simulink subsystem "station2a"  (R2024b)
settings: Solver=VariableStepAuto  StartTime=0.0  StopTime=10.0  RelTol=1e-3
undefined symbols (not defined in the file): DiscIntNeverNeededParam, h, R3, ResistanceM, Rt4, Ts, Zm
libraries: fl_lib x239, ee_lib x102, nesl_utility x83, simulink x6, simetran x1, powerlib_extras x1
(part 5 of 5)

== system station2a/Filters 60Hz5/tuned filter 13th ==
  Electrical Reference : fl_lib/Electrical/Electrical Elements/Electrical Reference
  Electrical Reference1 : fl_lib/Electrical/Electrical Elements/Electrical Reference
  Electrical Reference2 : fl_lib/Electrical/Electrical Elements/Electrical Reference
  Inductor : fl_lib/Electrical/Electrical Elements/Inductor  l=L1 H  r=R2 Ohm  g=1e-9 1/Ohm  i_specify=off  i_priority=None  i=0 A  i_nominal_specify=off  i_nominal_value=1  i_nominal_unit=A  v_specify=off  v_priority=None  v=0 V  v_nominal_specify=off  v_nominal_value=1  v_nominal_unit=V  i_L_specify=off  i_L_priority=High  i_L=0 A  i_L_nominal_specify=off  i_L_nominal_value=1  i_L_nominal_unit=A
  Inductor1 : fl_lib/Electrical/Electrical Elements/Inductor  l=L1 H  r=R2 Ohm  g=1e-9 1/Ohm  i_specify=off  i_priority=None  i=0 A  i_nominal_specify=off  i_nominal_value=1  i_nominal_unit=A  v_specify=off  v_priority=None  v=0 V  v_nominal_specify=off  v_nominal_value=1  v_nominal_unit=V  i_L_specify=off  i_L_priority=High  i_L=0 A  i_L_nominal_specify=off  i_L_nominal_value=1  i_L_nominal_unit=A
  Inductor2 : fl_lib/Electrical/Electrical Elements/Inductor  l=L1 H  r=R2 Ohm  g=1e-9 1/Ohm  i_specify=off  i_priority=None  i=0 A  i_nominal_specify=off  i_nominal_value=1  i_nominal_unit=A  v_specify=off  v_priority=None  v=0 V  v_nominal_specify=off  v_nominal_value=1  v_nominal_unit=V  i_L_specify=off  i_L_priority=High  i_L=0 A  i_L_nominal_specify=off  i_L_nominal_value=1  i_L_nominal_unit=A
  Phase Splitter : ee_lib/Connectors & References/Phase Splitter
  RC : fl_lib/Electrical/Electrical Elements/Capacitor  c=C1 F  r=0 Ohm  g=0 1/Ohm  i_specify=off  i_priority=None  i=0 A  i_nominal_specify=off  i_nominal_value=1  i_nominal_unit=A  v_specify=off  v_priority=None  v=0 V  v_nominal_specify=off  v_nominal_value=1  v_nominal_unit=V  vc_specify=off  vc_priority=High  vc=0 V  vc_nominal_specify=off  vc_nominal_value=1  vc_nominal_unit=V
  RC1 : fl_lib/Electrical/Electrical Elements/Capacitor  c=C1 F  r=0 Ohm  g=0 1/Ohm  i_specify=off  i_priority=None  i=0 A  i_nominal_specify=off  i_nominal_value=1  i_nominal_unit=A  v_specify=off  v_priority=None  v=0 V  v_nominal_specify=off  v_nominal_value=1  v_nominal_unit=V  vc_specify=off  vc_priority=High  vc=0 V  vc_nominal_specify=off  vc_nominal_value=1  vc_nominal_unit=V
  RC2 : fl_lib/Electrical/Electrical Elements/Capacitor  c=C1 F  r=0 Ohm  g=0 1/Ohm  i_specify=off  i_priority=None  i=0 A  i_nominal_specify=off  i_nominal_value=1  i_nominal_unit=A  v_specify=off  v_priority=None  v=0 V  v_nominal_specify=off  v_nominal_value=1  v_nominal_unit=V  vc_specify=off  vc_priority=High  vc=0 V  vc_nominal_specify=off  vc_nominal_value=1  vc_nominal_unit=V
  abc : PMIOPort  Side=Right
  connections:
  Inductor/LConn1 -- RC/RConn1
  Inductor/RConn1 -- Electrical Reference/LConn1
  RC1/RConn1 -- Inductor1/LConn1
  Inductor1/RConn1 -- Electrical Reference1/LConn1
  Inductor2/RConn1 -- Electrical Reference2/LConn1
  RC2/RConn1 -- Inductor2/LConn1
  Phase Splitter/RConn2 -- RC1/LConn1
  RC/LConn1 -- Phase Splitter/RConn1
  RC2/LConn1 -- Phase Splitter/RConn3
  Phase Splitter/LConn1 -- abc/RConn1

== system station2a/Filters 60Hz6/High-pass filter ==
  CC : fl_lib/Electrical/Electrical Elements/Capacitor  c=C1 F  r=0 Ohm  g=0 1/Ohm  i_specify=off  i_priority=None  i=0 A  i_nominal_specify=off  i_nominal_value=1  i_nominal_unit=A  v_specify=off  v_priority=None  v=0 V  v_nominal_specify=off  v_nominal_value=1  v_nominal_unit=V  vc_specify=off  vc_priority=High  vc=0 V  vc_nominal_specify=off  vc_nominal_value=1  vc_nominal_unit=V
  CC1 : fl_lib/Electrical/Electrical Elements/Capacitor  c=C1 F  r=0 Ohm  g=0 1/Ohm  i_specify=off  i_priority=None  i=0 A  i_nominal_specify=off  i_nominal_value=1  i_nominal_unit=A  v_specify=off  v_priority=None  v=0 V  v_nominal_specify=off  v_nominal_value=1  v_nominal_unit=V  vc_specify=off  vc_priority=High  vc=0 V  vc_nominal_specify=off  vc_nominal_value=1  vc_nominal_unit=V
  CC2 : fl_lib/Electrical/Electrical Elements/Capacitor  c=C1 F  r=0 Ohm  g=0 1/Ohm  i_specify=off  i_priority=None  i=0 A  i_nominal_specify=off  i_nominal_value=1  i_nominal_unit=A  v_specify=off  v_priority=None  v=0 V  v_nominal_specify=off  v_nominal_value=1  v_nominal_unit=V  vc_specify=off  vc_priority=High  vc=0 V  vc_nominal_specify=off  vc_nominal_value=1  vc_nominal_unit=V
  Electrical Reference : fl_lib/Electrical/Electrical Elements/Electrical Reference
  Electrical Reference1 : fl_lib/Electrical/Electrical Elements/Electrical Reference
  Electrical Reference2 : fl_lib/Electrical/Electrical Elements/Electrical Reference
  Phase Splitter : ee_lib/Connectors & References/Phase Splitter
  RL parallel : fl_lib/Electrical/Electrical Elements/Inductor  l=L2 H  r=0 Ohm  g=1/R3 1/Ohm  i_specify=off  i_priority=None  i=0 A  i_nominal_specify=off  i_nominal_value=1  i_nominal_unit=A  v_specify=off  v_priority=None  v=0 V  v_nominal_specify=off  v_nominal_value=1  v_nominal_unit=V  i_L_specify=off  i_L_priority=High  i_L=0 A  i_L_nominal_specify=off  i_L_nominal_value=1  i_L_nominal_unit=A
  RL parallel1 : fl_lib/Electrical/Electrical Elements/Inductor  l=L2 H  r=0 Ohm  g=1/R3 1/Ohm  i_specify=off  i_priority=None  i=0 A  i_nominal_specify=off  i_nominal_value=1  i_nominal_unit=A  v_specify=off  v_priority=None  v=0 V  v_nominal_specify=off  v_nominal_value=1  v_nominal_unit=V  i_L_specify=off  i_L_priority=High  i_L=0 A  i_L_nominal_specify=off  i_L_nominal_value=1  i_L_nominal_unit=A
  RL parallel2 : fl_lib/Electrical/Electrical Elements/Inductor  l=L2 H  r=0 Ohm  g=1/R3 1/Ohm  i_specify=off  i_priority=None  i=0 A  i_nominal_specify=off  i_nominal_value=1  i_nominal_unit=A  v_specify=off  v_priority=None  v=0 V  v_nominal_specify=off  v_nominal_value=1  v_nominal_unit=V  i_L_specify=off  i_L_priority=High  i_L=0 A  i_L_nominal_specify=off  i_L_nominal_value=1  i_L_nominal_unit=A
  abc : PMIOPort  Side=Right
  connections:
  CC2/RConn1 -- RL parallel2/LConn1
  RL parallel2/RConn1 -- Electrical Reference2/LConn1
  RL parallel1/RConn1 -- Electrical Reference1/LConn1
  CC1/RConn1 -- RL parallel1/LConn1
  RL parallel/RConn1 -- Electrical Reference/LConn1
  RL parallel/LConn1 -- CC/RConn1
  Phase Splitter/LConn1 -- abc/RConn1
  Phase Splitter/RConn2 -- CC1/LConn1
  CC/LConn1 -- Phase Splitter/RConn1
  CC2/LConn1 -- Phase Splitter/RConn3

== system station2a/Filters 60Hz6/tuned filter 11th ==
  Electrical Reference : fl_lib/Electrical/Electrical Elements/Electrical Reference
  Electrical Reference1 : fl_lib/Electrical/Electrical Elements/Electrical Reference
  Electrical Reference2 : fl_lib/Electrical/Electrical Elements/Electrical Reference
  Inductor : fl_lib/Electrical/Electrical Elements/Inductor  l=L1 H  r=R2 Ohm  g=1e-9 1/Ohm  i_specify=off  i_priority=None  i=0 A  i_nominal_specify=off  i_nominal_value=1  i_nominal_unit=A  v_specify=off  v_priority=None  v=0 V  v_nominal_specify=off  v_nominal_value=1  v_nominal_unit=V  i_L_specify=off  i_L_priority=High  i_L=0 A  i_L_nominal_specify=off  i_L_nominal_value=1  i_L_nominal_unit=A
  Inductor1 : fl_lib/Electrical/Electrical Elements/Inductor  l=L1 H  r=R2 Ohm  g=1e-9 1/Ohm  i_specify=off  i_priority=None  i=0 A  i_nominal_specify=off  i_nominal_value=1  i_nominal_unit=A  v_specify=off  v_priority=None  v=0 V  v_nominal_specify=off  v_nominal_value=1  v_nominal_unit=V  i_L_specify=off  i_L_priority=High  i_L=0 A  i_L_nominal_specify=off  i_L_nominal_value=1  i_L_nominal_unit=A
  Inductor2 : fl_lib/Electrical/Electrical Elements/Inductor  l=L1 H  r=R2 Ohm  g=1e-9 1/Ohm  i_specify=off  i_priority=None  i=0 A  i_nominal_specify=off  i_nominal_value=1  i_nominal_unit=A  v_specify=off  v_priority=None  v=0 V  v_nominal_specify=off  v_nominal_value=1  v_nominal_unit=V  i_L_specify=off  i_L_priority=High  i_L=0 A  i_L_nominal_specify=off  i_L_nominal_value=1  i_L_nominal_unit=A
  Phase Splitter : ee_lib/Connectors & References/Phase Splitter
  RC : fl_lib/Electrical/Electrical Elements/Capacitor  c=C1 F  r=0 Ohm  g=0 1/Ohm  i_specify=off  i_priority=None  i=0 A  i_nominal_specify=off  i_nominal_value=1  i_nominal_unit=A  v_specify=off  v_priority=None  v=0 V  v_nominal_specify=off  v_nominal_value=1  v_nominal_unit=V  vc_specify=off  vc_priority=High  vc=0 V  vc_nominal_specify=off  vc_nominal_value=1  vc_nominal_unit=V
  RC1 : fl_lib/Electrical/Electrical Elements/Capacitor  c=C1 F  r=0 Ohm  g=0 1/Ohm  i_specify=off  i_priority=None  i=0 A  i_nominal_specify=off  i_nominal_value=1  i_nominal_unit=A  v_specify=off  v_priority=None  v=0 V  v_nominal_specify=off  v_nominal_value=1  v_nominal_unit=V  vc_specify=off  vc_priority=High  vc=0 V  vc_nominal_specify=off  vc_nominal_value=1  vc_nominal_unit=V
  RC2 : fl_lib/Electrical/Electrical Elements/Capacitor  c=C1 F  r=0 Ohm  g=0 1/Ohm  i_specify=off  i_priority=None  i=0 A  i_nominal_specify=off  i_nominal_value=1  i_nominal_unit=A  v_specify=off  v_priority=None  v=0 V  v_nominal_specify=off  v_nominal_value=1  v_nominal_unit=V  vc_specify=off  vc_priority=High  vc=0 V  vc_nominal_specify=off  vc_nominal_value=1  vc_nominal_unit=V
  abc : PMIOPort  Side=Right
  connections:
  Inductor/LConn1 -- RC/RConn1
  Inductor/RConn1 -- Electrical Reference/LConn1
  RC1/RConn1 -- Inductor1/LConn1
  Inductor1/RConn1 -- Electrical Reference1/LConn1
  Inductor2/RConn1 -- Electrical Reference2/LConn1
  RC2/RConn1 -- Inductor2/LConn1
  Phase Splitter/RConn2 -- RC1/LConn1
  RC/LConn1 -- Phase Splitter/RConn1
  RC2/LConn1 -- Phase Splitter/RConn3
  Phase Splitter/LConn1 -- abc/RConn1

== system station2a/Filters 60Hz6/tuned filter 13th ==
  Electrical Reference : fl_lib/Electrical/Electrical Elements/Electrical Reference
  Electrical Reference1 : fl_lib/Electrical/Electrical Elements/Electrical Reference
  Electrical Reference2 : fl_lib/Electrical/Electrical Elements/Electrical Reference
  Inductor : fl_lib/Electrical/Electrical Elements/Inductor  l=L1 H  r=R2 Ohm  g=1e-9 1/Ohm  i_specify=off  i_priority=None  i=0 A  i_nominal_specify=off  i_nominal_value=1  i_nominal_unit=A  v_specify=off  v_priority=None  v=0 V  v_nominal_specify=off  v_nominal_value=1  v_nominal_unit=V  i_L_specify=off  i_L_priority=High  i_L=0 A  i_L_nominal_specify=off  i_L_nominal_value=1  i_L_nominal_unit=A
  Inductor1 : fl_lib/Electrical/Electrical Elements/Inductor  l=L1 H  r=R2 Ohm  g=1e-9 1/Ohm  i_specify=off  i_priority=None  i=0 A  i_nominal_specify=off  i_nominal_value=1  i_nominal_unit=A  v_specify=off  v_priority=None  v=0 V  v_nominal_specify=off  v_nominal_value=1  v_nominal_unit=V  i_L_specify=off  i_L_priority=High  i_L=0 A  i_L_nominal_specify=off  i_L_nominal_value=1  i_L_nominal_unit=A
  Inductor2 : fl_lib/Electrical/Electrical Elements/Inductor  l=L1 H  r=R2 Ohm  g=1e-9 1/Ohm  i_specify=off  i_priority=None  i=0 A  i_nominal_specify=off  i_nominal_value=1  i_nominal_unit=A  v_specify=off  v_priority=None  v=0 V  v_nominal_specify=off  v_nominal_value=1  v_nominal_unit=V  i_L_specify=off  i_L_priority=High  i_L=0 A  i_L_nominal_specify=off  i_L_nominal_value=1  i_L_nominal_unit=A
  Phase Splitter : ee_lib/Connectors & References/Phase Splitter
  RC : fl_lib/Electrical/Electrical Elements/Capacitor  c=C1 F  r=0 Ohm  g=0 1/Ohm  i_specify=off  i_priority=None  i=0 A  i_nominal_specify=off  i_nominal_value=1  i_nominal_unit=A  v_specify=off  v_priority=None  v=0 V  v_nominal_specify=off  v_nominal_value=1  v_nominal_unit=V  vc_specify=off  vc_priority=High  vc=0 V  vc_nominal_specify=off  vc_nominal_value=1  vc_nominal_unit=V
  RC1 : fl_lib/Electrical/Electrical Elements/Capacitor  c=C1 F  r=0 Ohm  g=0 1/Ohm  i_specify=off  i_priority=None  i=0 A  i_nominal_specify=off  i_nominal_value=1  i_nominal_unit=A  v_specify=off  v_priority=None  v=0 V  v_nominal_specify=off  v_nominal_value=1  v_nominal_unit=V  vc_specify=off  vc_priority=High  vc=0 V  vc_nominal_specify=off  vc_nominal_value=1  vc_nominal_unit=V
  RC2 : fl_lib/Electrical/Electrical Elements/Capacitor  c=C1 F  r=0 Ohm  g=0 1/Ohm  i_specify=off  i_priority=None  i=0 A  i_nominal_specify=off  i_nominal_value=1  i_nominal_unit=A  v_specify=off  v_priority=None  v=0 V  v_nominal_specify=off  v_nominal_value=1  v_nominal_unit=V  vc_specify=off  vc_priority=High  vc=0 V  vc_nominal_specify=off  vc_nominal_value=1  vc_nominal_unit=V
  abc : PMIOPort  Side=Right
  connections:
  Phase Splitter/LConn1 -- abc/RConn1
  RC2/LConn1 -- Phase Splitter/RConn3
  RC/LConn1 -- Phase Splitter/RConn1
  Phase Splitter/RConn2 -- RC1/LConn1
  RC2/RConn1 -- Inductor2/LConn1
  Inductor2/RConn1 -- Electrical Reference2/LConn1
  Inductor1/RConn1 -- Electrical Reference1/LConn1
  RC1/RConn1 -- Inductor1/LConn1
  Inductor/RConn1 -- Electrical Reference/LConn1
  Inductor/LConn1 -- RC/RConn1

== system station2a/Filters 60Hz7/High-pass filter ==
  CC : fl_lib/Electrical/Electrical Elements/Capacitor  c=C1 F  r=0 Ohm  g=0 1/Ohm  i_specify=off  i_priority=None  i=0 A  i_nominal_specify=off  i_nominal_value=1  i_nominal_unit=A  v_specify=off  v_priority=None  v=0 V  v_nominal_specify=off  v_nominal_value=1  v_nominal_unit=V  vc_specify=off  vc_priority=High  vc=0 V  vc_nominal_specify=off  vc_nominal_value=1  vc_nominal_unit=V
  CC1 : fl_lib/Electrical/Electrical Elements/Capacitor  c=C1 F  r=0 Ohm  g=0 1/Ohm  i_specify=off  i_priority=None  i=0 A  i_nominal_specify=off  i_nominal_value=1  i_nominal_unit=A  v_specify=off  v_priority=None  v=0 V  v_nominal_specify=off  v_nominal_value=1  v_nominal_unit=V  vc_specify=off  vc_priority=High  vc=0 V  vc_nominal_specify=off  vc_nominal_value=1  vc_nominal_unit=V
  CC2 : fl_lib/Electrical/Electrical Elements/Capacitor  c=C1 F  r=0 Ohm  g=0 1/Ohm  i_specify=off  i_priority=None  i=0 A  i_nominal_specify=off  i_nominal_value=1  i_nominal_unit=A  v_specify=off  v_priority=None  v=0 V  v_nominal_specify=off  v_nominal_value=1  v_nominal_unit=V  vc_specify=off  vc_priority=High  vc=0 V  vc_nominal_specify=off  vc_nominal_value=1  vc_nominal_unit=V
  Electrical Reference : fl_lib/Electrical/Electrical Elements/Electrical Reference
  Electrical Reference1 : fl_lib/Electrical/Electrical Elements/Electrical Reference
  Electrical Reference2 : fl_lib/Electrical/Electrical Elements/Electrical Reference
  Phase Splitter : ee_lib/Connectors & References/Phase Splitter
  RL parallel : fl_lib/Electrical/Electrical Elements/Inductor  l=L2 H  r=0 Ohm  g=1/R3 1/Ohm  i_specify=off  i_priority=None  i=0 A  i_nominal_specify=off  i_nominal_value=1  i_nominal_unit=A  v_specify=off  v_priority=None  v=0 V  v_nominal_specify=off  v_nominal_value=1  v_nominal_unit=V  i_L_specify=off  i_L_priority=High  i_L=0 A  i_L_nominal_specify=off  i_L_nominal_value=1  i_L_nominal_unit=A
  RL parallel1 : fl_lib/Electrical/Electrical Elements/Inductor  l=L2 H  r=0 Ohm  g=1/R3 1/Ohm  i_specify=off  i_priority=None  i=0 A  i_nominal_specify=off  i_nominal_value=1  i_nominal_unit=A  v_specify=off  v_priority=None  v=0 V  v_nominal_specify=off  v_nominal_value=1  v_nominal_unit=V  i_L_specify=off  i_L_priority=High  i_L=0 A  i_L_nominal_specify=off  i_L_nominal_value=1  i_L_nominal_unit=A
  RL parallel2 : fl_lib/Electrical/Electrical Elements/Inductor  l=L2 H  r=0 Ohm  g=1/R3 1/Ohm  i_specify=off  i_priority=None  i=0 A  i_nominal_specify=off  i_nominal_value=1  i_nominal_unit=A  v_specify=off  v_priority=None  v=0 V  v_nominal_specify=off  v_nominal_value=1  v_nominal_unit=V  i_L_specify=off  i_L_priority=High  i_L=0 A  i_L_nominal_specify=off  i_L_nominal_value=1  i_L_nominal_unit=A
  abc : PMIOPort  Side=Right
  connections:
  CC2/LConn1 -- Phase Splitter/RConn3
  CC/LConn1 -- Phase Splitter/RConn1
  Phase Splitter/RConn2 -- CC1/LConn1
  Phase Splitter/LConn1 -- abc/RConn1
  RL parallel/LConn1 -- CC/RConn1
  RL parallel/RConn1 -- Electrical Reference/LConn1
  CC1/RConn1 -- RL parallel1/LConn1
  RL parallel1/RConn1 -- Electrical Reference1/LConn1
  RL parallel2/RConn1 -- Electrical Reference2/LConn1
  CC2/RConn1 -- RL parallel2/LConn1

== system station2a/Filters 60Hz7/tuned filter 11th ==
  Electrical Reference : fl_lib/Electrical/Electrical Elements/Electrical Reference
  Electrical Reference1 : fl_lib/Electrical/Electrical Elements/Electrical Reference
  Electrical Reference2 : fl_lib/Electrical/Electrical Elements/Electrical Reference
  Inductor : fl_lib/Electrical/Electrical Elements/Inductor  l=L1 H  r=R2 Ohm  g=1e-9 1/Ohm  i_specify=off  i_priority=None  i=0 A  i_nominal_specify=off  i_nominal_value=1  i_nominal_unit=A  v_specify=off  v_priority=None  v=0 V  v_nominal_specify=off  v_nominal_value=1  v_nominal_unit=V  i_L_specify=off  i_L_priority=High  i_L=0 A  i_L_nominal_specify=off  i_L_nominal_value=1  i_L_nominal_unit=A
  Inductor1 : fl_lib/Electrical/Electrical Elements/Inductor  l=L1 H  r=R2 Ohm  g=1e-9 1/Ohm  i_specify=off  i_priority=None  i=0 A  i_nominal_specify=off  i_nominal_value=1  i_nominal_unit=A  v_specify=off  v_priority=None  v=0 V  v_nominal_specify=off  v_nominal_value=1  v_nominal_unit=V  i_L_specify=off  i_L_priority=High  i_L=0 A  i_L_nominal_specify=off  i_L_nominal_value=1  i_L_nominal_unit=A
  Inductor2 : fl_lib/Electrical/Electrical Elements/Inductor  l=L1 H  r=R2 Ohm  g=1e-9 1/Ohm  i_specify=off  i_priority=None  i=0 A  i_nominal_specify=off  i_nominal_value=1  i_nominal_unit=A  v_specify=off  v_priority=None  v=0 V  v_nominal_specify=off  v_nominal_value=1  v_nominal_unit=V  i_L_specify=off  i_L_priority=High  i_L=0 A  i_L_nominal_specify=off  i_L_nominal_value=1  i_L_nominal_unit=A
  Phase Splitter : ee_lib/Connectors & References/Phase Splitter
  RC : fl_lib/Electrical/Electrical Elements/Capacitor  c=C1 F  r=0 Ohm  g=0 1/Ohm  i_specify=off  i_priority=None  i=0 A  i_nominal_specify=off  i_nominal_value=1  i_nominal_unit=A  v_specify=off  v_priority=None  v=0 V  v_nominal_specify=off  v_nominal_value=1  v_nominal_unit=V  vc_specify=off  vc_priority=High  vc=0 V  vc_nominal_specify=off  vc_nominal_value=1  vc_nominal_unit=V
  RC1 : fl_lib/Electrical/Electrical Elements/Capacitor  c=C1 F  r=0 Ohm  g=0 1/Ohm  i_specify=off  i_priority=None  i=0 A  i_nominal_specify=off  i_nominal_value=1  i_nominal_unit=A  v_specify=off  v_priority=None  v=0 V  v_nominal_specify=off  v_nominal_value=1  v_nominal_unit=V  vc_specify=off  vc_priority=High  vc=0 V  vc_nominal_specify=off  vc_nominal_value=1  vc_nominal_unit=V
  RC2 : fl_lib/Electrical/Electrical Elements/Capacitor  c=C1 F  r=0 Ohm  g=0 1/Ohm  i_specify=off  i_priority=None  i=0 A  i_nominal_specify=off  i_nominal_value=1  i_nominal_unit=A  v_specify=off  v_priority=None  v=0 V  v_nominal_specify=off  v_nominal_value=1  v_nominal_unit=V  vc_specify=off  vc_priority=High  vc=0 V  vc_nominal_specify=off  vc_nominal_value=1  vc_nominal_unit=V
  abc : PMIOPort  Side=Right
  connections:
  Phase Splitter/LConn1 -- abc/RConn1
  RC2/LConn1 -- Phase Splitter/RConn3
  RC/LConn1 -- Phase Splitter/RConn1
  Phase Splitter/RConn2 -- RC1/LConn1
  RC2/RConn1 -- Inductor2/LConn1
  Inductor2/RConn1 -- Electrical Reference2/LConn1
  Inductor1/RConn1 -- Electrical Reference1/LConn1
  RC1/RConn1 -- Inductor1/LConn1
  Inductor/RConn1 -- Electrical Reference/LConn1
  Inductor/LConn1 -- RC/RConn1

== system station2a/Filters 60Hz7/tuned filter 13th ==
  Electrical Reference : fl_lib/Electrical/Electrical Elements/Electrical Reference
  Electrical Reference1 : fl_lib/Electrical/Electrical Elements/Electrical Reference
  Electrical Reference2 : fl_lib/Electrical/Electrical Elements/Electrical Reference
  Inductor : fl_lib/Electrical/Electrical Elements/Inductor  l=L1 H  r=R2 Ohm  g=1e-9 1/Ohm  i_specify=off  i_priority=None  i=0 A  i_nominal_specify=off  i_nominal_value=1  i_nominal_unit=A  v_specify=off  v_priority=None  v=0 V  v_nominal_specify=off  v_nominal_value=1  v_nominal_unit=V  i_L_specify=off  i_L_priority=High  i_L=0 A  i_L_nominal_specify=off  i_L_nominal_value=1  i_L_nominal_unit=A
  Inductor1 : fl_lib/Electrical/Electrical Elements/Inductor  l=L1 H  r=R2 Ohm  g=1e-9 1/Ohm  i_specify=off  i_priority=None  i=0 A  i_nominal_specify=off  i_nominal_value=1  i_nominal_unit=A  v_specify=off  v_priority=None  v=0 V  v_nominal_specify=off  v_nominal_value=1  v_nominal_unit=V  i_L_specify=off  i_L_priority=High  i_L=0 A  i_L_nominal_specify=off  i_L_nominal_value=1  i_L_nominal_unit=A
  Inductor2 : fl_lib/Electrical/Electrical Elements/Inductor  l=L1 H  r=R2 Ohm  g=1e-9 1/Ohm  i_specify=off  i_priority=None  i=0 A  i_nominal_specify=off  i_nominal_value=1  i_nominal_unit=A  v_specify=off  v_priority=None  v=0 V  v_nominal_specify=off  v_nominal_value=1  v_nominal_unit=V  i_L_specify=off  i_L_priority=High  i_L=0 A  i_L_nominal_specify=off  i_L_nominal_value=1  i_L_nominal_unit=A
  Phase Splitter : ee_lib/Connectors & References/Phase Splitter
  RC : fl_lib/Electrical/Electrical Elements/Capacitor  c=C1 F  r=0 Ohm  g=0 1/Ohm  i_specify=off  i_priority=None  i=0 A  i_nominal_specify=off  i_nominal_value=1  i_nominal_unit=A  v_specify=off  v_priority=None  v=0 V  v_nominal_specify=off  v_nominal_value=1  v_nominal_unit=V  vc_specify=off  vc_priority=High  vc=0 V  vc_nominal_specify=off  vc_nominal_value=1  vc_nominal_unit=V
  RC1 : fl_lib/Electrical/Electrical Elements/Capacitor  c=C1 F  r=0 Ohm  g=0 1/Ohm  i_specify=off  i_priority=None  i=0 A  i_nominal_specify=off  i_nominal_value=1  i_nominal_unit=A  v_specify=off  v_priority=None  v=0 V  v_nominal_specify=off  v_nominal_value=1  v_nominal_unit=V  vc_specify=off  vc_priority=High  vc=0 V  vc_nominal_specify=off  vc_nominal_value=1  vc_nominal_unit=V
  RC2 : fl_lib/Electrical/Electrical Elements/Capacitor  c=C1 F  r=0 Ohm  g=0 1/Ohm  i_specify=off  i_priority=None  i=0 A  i_nominal_specify=off  i_nominal_value=1  i_nominal_unit=A  v_specify=off  v_priority=None  v=0 V  v_nominal_specify=off  v_nominal_value=1  v_nominal_unit=V  vc_specify=off  vc_priority=High  vc=0 V  vc_nominal_specify=off  vc_nominal_value=1  vc_nominal_unit=V
  abc : PMIOPort  Side=Right
  connections:
  Inductor/LConn1 -- RC/RConn1
  Inductor/RConn1 -- Electrical Reference/LConn1
  RC1/RConn1 -- Inductor1/LConn1
  Inductor1/RConn1 -- Electrical Reference1/LConn1
  Inductor2/RConn1 -- Electrical Reference2/LConn1
  RC2/RConn1 -- Inductor2/LConn1
  Phase Splitter/RConn2 -- RC1/LConn1
  RC/LConn1 -- Phase Splitter/RConn1
  RC2/LConn1 -- Phase Splitter/RConn3
  Phase Splitter/LConn1 -- abc/RConn1

== system station2a/Half-DPL1ph1/Simscape ==
  Electrical Reference1 : fl_lib/Electrical/Electrical Elements/Electrical Reference
  PS-S : nesl_utility/PS-Simulink Converter  PhysicalDomain=network_engine_domain  SubClassName=ps_output  LeftPortType=input  RightPortType=output  PseudoPeriodic=off  Frequencies=[]  VectorFormat=1-D array  Unit=V  AffineConversion=off
  Voltage Sensor : fl_lib/Electrical/Electrical Sensors/Voltage Sensor
  V : PMIOPort  Side=Left
  Out : Outport  VectorParamsAs1DForOutWhenUnconnected=off
  wires:
  PS-S/1 -> Out/1  "voltage"
  connections:
  Electrical Reference1/LConn1 -- Voltage Sensor/RConn2
  V/RConn1 -- Voltage Sensor/LConn1
  PS-S/LConn1 -- Voltage Sensor/RConn1

== system station2a/Half-DPL1ph1/Voltage Source ==
  I : Inport
  Controlled Current Source1 : fl_lib/Electrical/Electrical Sources/Controlled Current Source
  Simulink-PS Converter : nesl_utility/Simulink-PS Converter  PhysicalDomain=network_engine_domain  SubClassName=ps_input  LeftPortType=input  RightPortType=output  PseudoPeriodic=off  Frequencies=[]  NoiseDistribution=none  NoiseParameters=[]  Unit=1  AffineConversion=off  FilteringAndDerivatives=zero  SimscapeFilterOrder=1  InputFilterTimeConstant=.001  UdotUserProvided=0
  + : PMIOPort  Side=Right
  - : PMIOPort  Port=2  Side=Right
  wires:
  I/1 -> Simulink-PS Converter/1
  connections:
  Controlled Current Source1/LConn1 -- +/RConn1
  Controlled Current Source1/RConn2 -- -/RConn1
  Controlled Current Source1/RConn1 -- Simulink-PS Converter/RConn1

== system station2a/Half-DPL1ph1/dplmodel ==
  v : Inport
  hist_in : Inport  Port=2
  (1+h)/Z : Gain  Gain=(1+h)./(Zm+Rt4)  SaturateOnIntegerOverflow=on  OutDataTypeStr=Inherit: Same as input  ParamDataTypeStr=Inherit: Same as input
  Gain4 : Gain  Gain=(1+h)/2  SaturateOnIntegerOverflow=on  OutDataTypeStr=Inherit: Same as input  ParamDataTypeStr=Inherit: Same as input
  Gain6 : Gain  Gain=(1-h)/2  SaturateOnIntegerOverflow=on  OutDataTypeStr=Inherit: Same as input  ParamDataTypeStr=Inherit: Same as input
  Gain9 : Gain  Gain=h  SaturateOnIntegerOverflow=on  OutDataTypeStr=Inherit: Same as input  ParamDataTypeStr=Inherit: Same as input
  Sum1 : Sum  Inputs=-+  InputSameDT=on  SaturateOnIntegerOverflow=on  OutDataTypeStr=Inherit: Same as first input
  Sum3 : Sum  InputSameDT=on  SaturateOnIntegerOverflow=on  OutDataTypeStr=Inherit: Same as first input
  derlay : Subsystem
  i : Outport  InitialOutput=0  VectorParamsAs1DForOutWhenUnconnected=off
  hist_out : Outport  Port=2  VectorParamsAs1DForOutWhenUnconnected=off
  wires:
  Sum1/1 -> derlay/1(In1)
  derlay/1(Out1) -> Gain6/1, Gain4/1
  hist_in/1 -> Sum3/2
  Gain6/1 -> Sum3/1
  (1+h)/Z/1 -> Sum1/2
  Gain9/1 -> Sum1/1
  Gain4/1 -> hist_out/1
  v/1 -> (1+h)/Z/1
  Sum3/1 -> Gain9/1, i/1

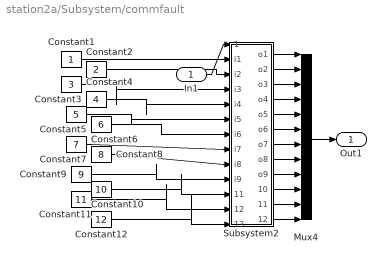
== system station2a/Subsystem/commfault ==
  In1 : Inport
  Constant1 : Constant
  Constant10 : Constant  Value=10
  Constant11 : Constant  Value=11
  Constant12 : Constant  Value=12
  Constant2 : Constant  Value=2
  Constant3 : Constant  Value=3
  Constant4 : Constant  Value=4
  Constant5 : Constant  Value=5
  Constant6 : Constant  Value=6
  Constant7 : Constant  Value=7
  Constant8 : Constant  Value=8
  Constant9 : Constant  Value=9
  Mux4 : Mux  Inputs=12
  Subsystem2 : Subsystem
  Out1 : Outport
  wires:
  Mux4/1 -> Out1/1
  In1/1 -> Subsystem2/1(In1)
  Subsystem2/12(o12) -> Mux4/12
  Subsystem2/11(o11) -> Mux4/11
  Subsystem2/10(o10) -> Mux4/10
  Subsystem2/9(o9) -> Mux4/9
  Subsystem2/8(o8) -> Mux4/8
  Subsystem2/7(o7) -> Mux4/7
  Subsystem2/6(o6) -> Mux4/6
  Subsystem2/5(o5) -> Mux4/5
  Subsystem2/4(o4) -> Mux4/4
  Subsystem2/3(o3) -> Mux4/3
  Subsystem2/2(o2) -> Mux4/2
  Subsystem2/1(o1) -> Mux4/1
  Constant12/1 -> Subsystem2/13(i12)
  Constant11/1 -> Subsystem2/12(i11)
  Constant10/1 -> Subsystem2/11(i10)
  Constant9/1 -> Subsystem2/10(i9)
  Constant8/1 -> Subsystem2/9(i8)
  Constant7/1 -> Subsystem2/8(i7)
  Constant6/1 -> Subsystem2/7(i6)
  Constant5/1 -> Subsystem2/6(i5)
  Constant4/1 -> Subsystem2/5(i4)
  Constant3/1 -> Subsystem2/4(i3)
  Constant2/1 -> Subsystem2/3(i2)
  Constant1/1 -> Subsystem2/2(i1)

== system station2a/Half-DPL1ph1/dplmodel/derlay ==
  In1 : Inport
  Add : Sum
  Delay1 : Delay  DelayLength=delay(1)
  Gain : Gain  Gain=remd
  Gain1 : Gain  Gain=1-remd
  Unit Delay1 : UnitDelay  SampleTime=Ts  HasFrameUpgradeWarning=on
  Out1 : Outport
  wires:
  Delay1/1 -> Unit Delay1/1, Gain1/1
  Add/1 -> Out1/1
  Unit Delay1/1 -> Gain/1
  Gain1/1 -> Add/2
  Gain/1 -> Add/1
  In1/1 -> Delay1/1

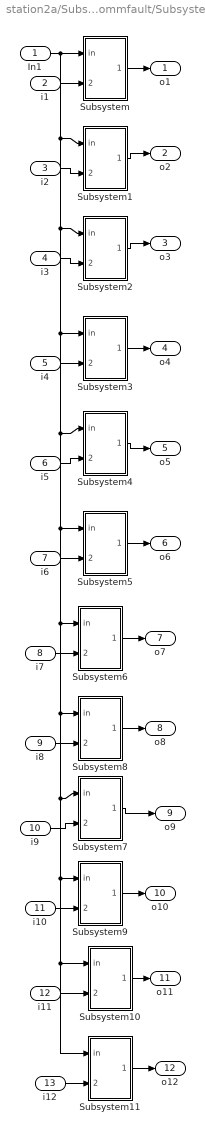
== system station2a/Subsystem/commfault/Subsystem2 ==
  In1 : Inport
  i1 : Inport  Port=2
  i2 : Inport  Port=3
  i3 : Inport  Port=4
  i4 : Inport  Port=5
  i5 : Inport  Port=6
  i6 : Inport  Port=7
  i7 : Inport  Port=8
  i8 : Inport  Port=9
  i9 : Inport  Port=10
  i10 : Inport  Port=11
  i11 : Inport  Port=12
  i12 : Inport  Port=13
  Subsystem : Subsystem
  Subsystem1 : Subsystem
  Subsystem10 : Subsystem
  Subsystem11 : Subsystem
  Subsystem2 : Subsystem
  Subsystem3 : Subsystem
  Subsystem4 : Subsystem
  Subsystem5 : Subsystem
  Subsystem6 : Subsystem
  Subsystem7 : Subsystem
  Subsystem8 : Subsystem
  Subsystem9 : Subsystem
  o1 : Outport
  o2 : Outport  Port=2
  o3 : Outport  Port=3
  o4 : Outport  Port=4
  o5 : Outport  Port=5
  o6 : Outport  Port=6
  o7 : Outport  Port=7
  o8 : Outport  Port=8
  o9 : Outport  Port=9
  o10 : Outport  Port=10
  o11 : Outport  Port=11
  o12 : Outport  Port=12
  wires:
  Subsystem11/1(Out1) -> o12/1
  Subsystem10/1(Out1) -> o11/1
  Subsystem9/1(Out1) -> o10/1
  Subsystem7/1(Out1) -> o9/1
  Subsystem8/1(Out1) -> o8/1
  Subsystem6/1(Out1) -> o7/1
  Subsystem5/1(Out1) -> o6/1
  Subsystem4/1(Out1) -> o5/1
  Subsystem3/1(Out1) -> o4/1
  Subsystem2/1(Out1) -> o3/1
  i12/1 -> Subsystem11/2(ind)
  i11/1 -> Subsystem10/2(ind)
  i10/1 -> Subsystem9/2(ind)
  i9/1 -> Subsystem7/2(ind)
  i8/1 -> Subsystem8/2(ind)
  i7/1 -> Subsystem6/2(ind)
  i6/1 -> Subsystem5/2(ind)
  i5/1 -> Subsystem4/2(ind)
  i4/1 -> Subsystem3/2(ind)
  i3/1 -> Subsystem2/2(ind)
  i2/1 -> Subsystem1/2(ind)
  Subsystem1/1(Out1) -> o2/1
  i1/1 -> Subsystem/2(ind)
  Subsystem/1(Out1) -> o1/1
  In1/1 -> Subsystem1/1(in), Subsystem2/1(in), Subsystem3/1(in), Subsystem4/1(in), Subsystem5/1(in), Subsystem6/1(in), Subsystem8/1(in), Subsystem7/1(in), Subsystem9/1(in), Subsystem11/1(in), Subsystem10/1(in), Subsystem/1(in)

== system station2a/Subsystem/commfault/Subsystem2/Subsystem ==
  in : Inport
  ind : Inport  Port=2
  Constant3 : Constant  Value=[1 0]
  Data Type Conversion : DataTypeConversion  OutDataTypeStr=double  SaturateOnIntegerOverflow=off  RndMeth=Floor
  Relational Operator : RelationalOperator  Operator===  OutDataTypeStr=boolean  InputSameDT=off
  Selector1 : Selector  IndexMode=Zero-based  InputPortWidth=2  IndexOptions=Index vector (port)  Indices=1  OutputSizes=1
  Out1 : Outport
  wires:
  Data Type Conversion/1 -> Selector1/2
  Relational Operator/1 -> Data Type Conversion/1
  Constant3/1 -> Selector1/1
  Selector1/1 -> Out1/1
  ind/1 -> Relational Operator/2
  in/1 -> Relational Operator/1

== system station2a/Subsystem/commfault/Subsystem2/Subsystem1 ==
  in : Inport
  ind : Inport  Port=2
  Constant3 : Constant  Value=[1 0]
  Data Type Conversion : DataTypeConversion  OutDataTypeStr=double  SaturateOnIntegerOverflow=off  RndMeth=Floor
  Relational Operator : RelationalOperator  Operator===  OutDataTypeStr=boolean  InputSameDT=off
  Selector1 : Selector  IndexMode=Zero-based  InputPortWidth=2  IndexOptions=Index vector (port)  Indices=1  OutputSizes=1
  Out1 : Outport
  wires:
  in/1 -> Relational Operator/1
  ind/1 -> Relational Operator/2
  Selector1/1 -> Out1/1
  Constant3/1 -> Selector1/1
  Relational Operator/1 -> Data Type Conversion/1
  Data Type Conversion/1 -> Selector1/2

== system station2a/Subsystem/commfault/Subsystem2/Subsystem10 ==
  in : Inport
  ind : Inport  Port=2
  Constant3 : Constant  Value=[1 0]
  Data Type Conversion : DataTypeConversion  OutDataTypeStr=double  SaturateOnIntegerOverflow=off  RndMeth=Floor
  Relational Operator : RelationalOperator  Operator===  OutDataTypeStr=boolean  InputSameDT=off
  Selector1 : Selector  IndexMode=Zero-based  InputPortWidth=2  IndexOptions=Index vector (port)  Indices=1  OutputSizes=1
  Out1 : Outport
  wires:
  in/1 -> Relational Operator/1
  ind/1 -> Relational Operator/2
  Selector1/1 -> Out1/1
  Constant3/1 -> Selector1/1
  Relational Operator/1 -> Data Type Conversion/1
  Data Type Conversion/1 -> Selector1/2

== system station2a/Subsystem/commfault/Subsystem2/Subsystem11 ==
  in : Inport
  ind : Inport  Port=2
  Constant3 : Constant  Value=[1 0]
  Data Type Conversion : DataTypeConversion  OutDataTypeStr=double  SaturateOnIntegerOverflow=off  RndMeth=Floor
  Relational Operator : RelationalOperator  Operator===  OutDataTypeStr=boolean  InputSameDT=off
  Selector1 : Selector  IndexMode=Zero-based  InputPortWidth=2  IndexOptions=Index vector (port)  Indices=1  OutputSizes=1
  Out1 : Outport
  wires:
  Data Type Conversion/1 -> Selector1/2
  Relational Operator/1 -> Data Type Conversion/1
  Constant3/1 -> Selector1/1
  Selector1/1 -> Out1/1
  ind/1 -> Relational Operator/2
  in/1 -> Relational Operator/1

== system station2a/Subsystem/commfault/Subsystem2/Subsystem2 ==
  in : Inport
  ind : Inport  Port=2
  Constant3 : Constant  Value=[1 0]
  Data Type Conversion : DataTypeConversion  OutDataTypeStr=double  SaturateOnIntegerOverflow=off  RndMeth=Floor
  Relational Operator : RelationalOperator  Operator===  OutDataTypeStr=boolean  InputSameDT=off
  Selector1 : Selector  IndexMode=Zero-based  InputPortWidth=2  IndexOptions=Index vector (port)  Indices=1  OutputSizes=1
  Out1 : Outport
  wires:
  Data Type Conversion/1 -> Selector1/2
  Relational Operator/1 -> Data Type Conversion/1
  Constant3/1 -> Selector1/1
  Selector1/1 -> Out1/1
  ind/1 -> Relational Operator/2
  in/1 -> Relational Operator/1

== system station2a/Subsystem/commfault/Subsystem2/Subsystem3 ==
  in : Inport
  ind : Inport  Port=2
  Constant3 : Constant  Value=[1 0]
  Data Type Conversion : DataTypeConversion  OutDataTypeStr=double  SaturateOnIntegerOverflow=off  RndMeth=Floor
  Relational Operator : RelationalOperator  Operator===  OutDataTypeStr=boolean  InputSameDT=off
  Selector1 : Selector  IndexMode=Zero-based  InputPortWidth=2  IndexOptions=Index vector (port)  Indices=1  OutputSizes=1
  Out1 : Outport
  wires:
  in/1 -> Relational Operator/1
  ind/1 -> Relational Operator/2
  Selector1/1 -> Out1/1
  Constant3/1 -> Selector1/1
  Relational Operator/1 -> Data Type Conversion/1
  Data Type Conversion/1 -> Selector1/2

== system station2a/Subsystem/commfault/Subsystem2/Subsystem4 ==
  in : Inport
  ind : Inport  Port=2
  Constant3 : Constant  Value=[1 0]
  Data Type Conversion : DataTypeConversion  OutDataTypeStr=double  SaturateOnIntegerOverflow=off  RndMeth=Floor
  Relational Operator : RelationalOperator  Operator===  OutDataTypeStr=boolean  InputSameDT=off
  Selector1 : Selector  IndexMode=Zero-based  InputPortWidth=2  IndexOptions=Index vector (port)  Indices=1  OutputSizes=1
  Out1 : Outport
  wires:
  Data Type Conversion/1 -> Selector1/2
  Relational Operator/1 -> Data Type Conversion/1
  Constant3/1 -> Selector1/1
  Selector1/1 -> Out1/1
  ind/1 -> Relational Operator/2
  in/1 -> Relational Operator/1

== system station2a/Subsystem/commfault/Subsystem2/Subsystem5 ==
  in : Inport
  ind : Inport  Port=2
  Constant3 : Constant  Value=[1 0]
  Data Type Conversion : DataTypeConversion  OutDataTypeStr=double  SaturateOnIntegerOverflow=off  RndMeth=Floor
  Relational Operator : RelationalOperator  Operator===  OutDataTypeStr=boolean  InputSameDT=off
  Selector1 : Selector  IndexMode=Zero-based  InputPortWidth=2  IndexOptions=Index vector (port)  Indices=1  OutputSizes=1
  Out1 : Outport
  wires:
  in/1 -> Relational Operator/1
  ind/1 -> Relational Operator/2
  Selector1/1 -> Out1/1
  Constant3/1 -> Selector1/1
  Relational Operator/1 -> Data Type Conversion/1
  Data Type Conversion/1 -> Selector1/2

== system station2a/Subsystem/commfault/Subsystem2/Subsystem6 ==
  in : Inport
  ind : Inport  Port=2
  Constant3 : Constant  Value=[1 0]
  Data Type Conversion : DataTypeConversion  OutDataTypeStr=double  SaturateOnIntegerOverflow=off  RndMeth=Floor
  Relational Operator : RelationalOperator  Operator===  OutDataTypeStr=boolean  InputSameDT=off
  Selector1 : Selector  IndexMode=Zero-based  InputPortWidth=2  IndexOptions=Index vector (port)  Indices=1  OutputSizes=1
  Out1 : Outport
  wires:
  Data Type Conversion/1 -> Selector1/2
  Relational Operator/1 -> Data Type Conversion/1
  Constant3/1 -> Selector1/1
  Selector1/1 -> Out1/1
  ind/1 -> Relational Operator/2
  in/1 -> Relational Operator/1

== system station2a/Subsystem/commfault/Subsystem2/Subsystem7 ==
  in : Inport
  ind : Inport  Port=2
  Constant3 : Constant  Value=[1 0]
  Data Type Conversion : DataTypeConversion  OutDataTypeStr=double  SaturateOnIntegerOverflow=off  RndMeth=Floor
  Relational Operator : RelationalOperator  Operator===  OutDataTypeStr=boolean  InputSameDT=off
  Selector1 : Selector  IndexMode=Zero-based  InputPortWidth=2  IndexOptions=Index vector (port)  Indices=1  OutputSizes=1
  Out1 : Outport
  wires:
  in/1 -> Relational Operator/1
  ind/1 -> Relational Operator/2
  Selector1/1 -> Out1/1
  Constant3/1 -> Selector1/1
  Relational Operator/1 -> Data Type Conversion/1
  Data Type Conversion/1 -> Selector1/2

== system station2a/Subsystem/commfault/Subsystem2/Subsystem8 ==
  in : Inport
  ind : Inport  Port=2
  Constant3 : Constant  Value=[1 0]
  Data Type Conversion : DataTypeConversion  OutDataTypeStr=double  SaturateOnIntegerOverflow=off  RndMeth=Floor
  Relational Operator : RelationalOperator  Operator===  OutDataTypeStr=boolean  InputSameDT=off
  Selector1 : Selector  IndexMode=Zero-based  InputPortWidth=2  IndexOptions=Index vector (port)  Indices=1  OutputSizes=1
  Out1 : Outport
  wires:
  Data Type Conversion/1 -> Selector1/2
  Relational Operator/1 -> Data Type Conversion/1
  Constant3/1 -> Selector1/1
  Selector1/1 -> Out1/1
  ind/1 -> Relational Operator/2
  in/1 -> Relational Operator/1

== system station2a/Subsystem/commfault/Subsystem2/Subsystem9 ==
  in : Inport
  ind : Inport  Port=2
  Constant3 : Constant  Value=[1 0]
  Data Type Conversion : DataTypeConversion  OutDataTypeStr=double  SaturateOnIntegerOverflow=off  RndMeth=Floor
  Relational Operator : RelationalOperator  Operator===  OutDataTypeStr=boolean  InputSameDT=off
  Selector1 : Selector  IndexMode=Zero-based  InputPortWidth=2  IndexOptions=Index vector (port)  Indices=1  OutputSizes=1
  Out1 : Outport
  wires:
  Data Type Conversion/1 -> Selector1/2
  Relational Operator/1 -> Data Type Conversion/1
  Constant3/1 -> Selector1/1
  Selector1/1 -> Out1/1
  ind/1 -> Relational Operator/2
  in/1 -> Relational Operator/1
